simulink model "model"  (R2014b)
settings: Solver=ode45  StartTime=0.0  StopTime=10.0  RelTol=1e-3
settings Model: Creator=Dyzio  LastModifiedBy=Dyzio

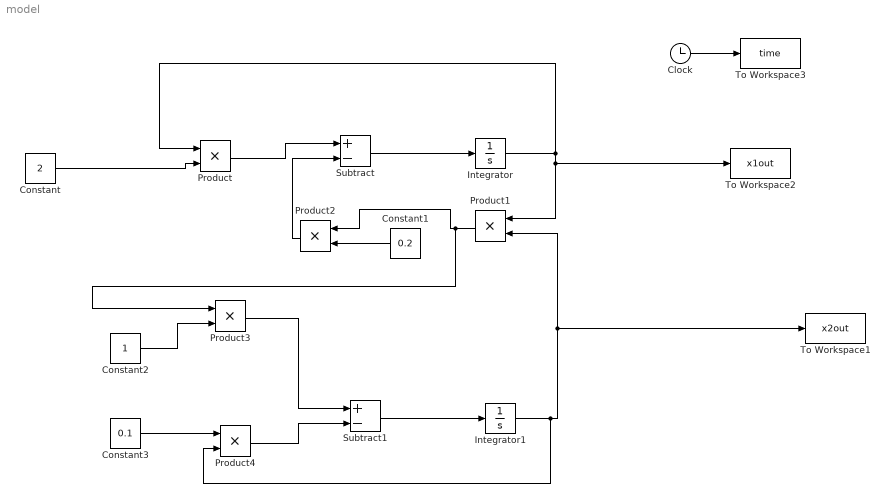
== system model ==
  Clock : Clock
  Constant : Constant  Value=2
  Constant1 : Constant  Value=0.2
  Constant2 : Constant
  Constant3 : Constant  Value=0.1
  Integrator : Integrator  InitialCondition=50
  Integrator1 : Integrator  InitialCondition=100
  Product{,1..4} (5 alike) : Product
  Subtract : Sum  Inputs=+-
  Subtract1 : Sum  Inputs=+-
  To Workspace1 : ToWorkspace  VariableName=x2out  SampleTime=-1
  To Workspace2 : ToWorkspace  VariableName=x1out  SampleTime=-1
  To Workspace3 : ToWorkspace  VariableName=time  SampleTime=-1
  wires:
  Subtract/1 -> Integrator/1
  Subtract1/1 -> Integrator1/1
  Constant/1 -> Product/2
  Integrator1/1 -> Product4/2, Product1/2, To Workspace1/1
  Product1/1 -> Product3/1, Product2/1
  Constant1/1 -> Product2/2
  Product/1 -> Subtract/1
  Product2/1 -> Subtract/2
  Constant2/1 -> Product3/2
  Constant3/1 -> Product4/1
  Product3/1 -> Subtract1/1
  Product4/1 -> Subtract1/2
  Integrator/1 -> To Workspace2/1, Product1/1, Product/1
  Clock/1 -> To Workspace3/1
